simulink model "nano_distribution_distiller_controller_ver1"  (R2021a)
settings: Solver=VariableStepAuto  StartTime=0.0  StopTime=10.0  RelTol=1e-3
libraries: arduinolib x14
settings Model: Creator=Intuito_PC  LastModifiedBy=Intuito_PC

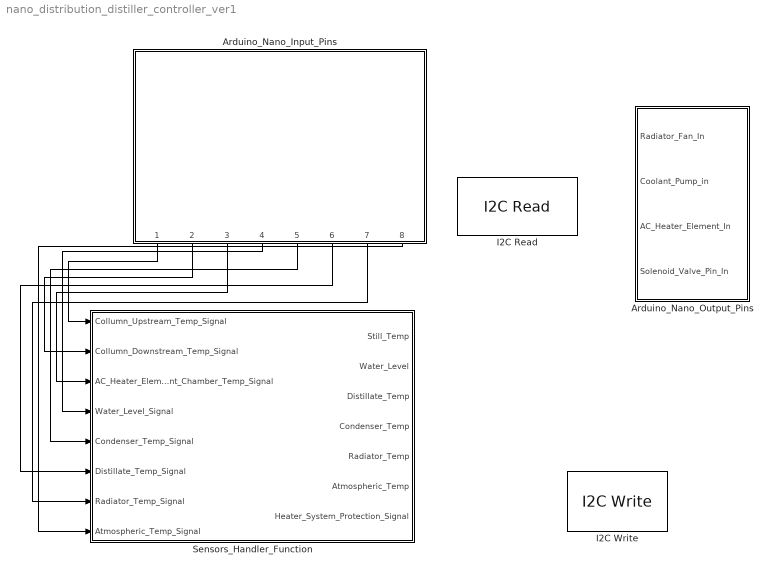
== system nano_distribution_distiller_controller_ver1 ==
  Arduino_Nano_Input_Pins : Subsystem
  Arduino_Nano_Output_Pins : Subsystem
  I2C Read : arduinolib/I2C Read  I2CModule=0  Mode=Master  SlaveAddress=10  SlaveByteOrder=BigEndian  Direction=Receiver  RegisterAddressMode=on  RegisterAddress=0  SlaveDataType=uint8  DataLength=1  NoAck=off  RepeatedStart=off  OutputStatus=off  blockPlatform=ARDUINO  SampleTime=0.25
      settings: SourceProductBaseCode=ARDUINO
  I2C Write : arduinolib/I2C Write  I2CModule=0  Mode=Master  SlaveAddress=10  SlaveByteOrder=BigEndian  Direction=Transmitter  RegisterAddressMode=on  RegisterAddress=0  SlaveDataType=uint8  DataLength=1  NoAck=off  RepeatedStart=off  OutputStatus=off  blockPlatform=ARDUINO
      settings: SourceProductBaseCode=ARDUINO
  Sensors_Handler_Function : Subsystem
  wires:
  Arduino_Nano_Input_Pins/8(Atmospheric_Temp_Signal) -> Sensors_Handler_Function/8(Atmospheric_Temp_Signal)
  Arduino_Nano_Input_Pins/7(Radiator_Temp_Signal) -> Sensors_Handler_Function/7(Radiator_Temp_Signal)
  Arduino_Nano_Input_Pins/3(AC_Heater_Element_Chamber_Temp_Signal) -> Sensors_Handler_Function/3(AC_Heater_Element_Chamber_Temp_Signal)
  Arduino_Nano_Input_Pins/1(Collumn_Upstream_Temp_Signal) -> Sensors_Handler_Function/1(Collumn_Upstream_Temp_Signal)
  Arduino_Nano_Input_Pins/2(Collumn_Downstream_Temp_Signal) -> Sensors_Handler_Function/2(Collumn_Downstream_Temp_Signal)
  Arduino_Nano_Input_Pins/6(Distillate_Temp_Signal) -> Sensors_Handler_Function/6(Distillate_Temp_Signal)
  Arduino_Nano_Input_Pins/5(Condenser_Temp_Signal) -> Sensors_Handler_Function/5(Condenser_Temp_Signal)
  Arduino_Nano_Input_Pins/4(Water_Level_Signal) -> Sensors_Handler_Function/4(Water_Level_Signal)

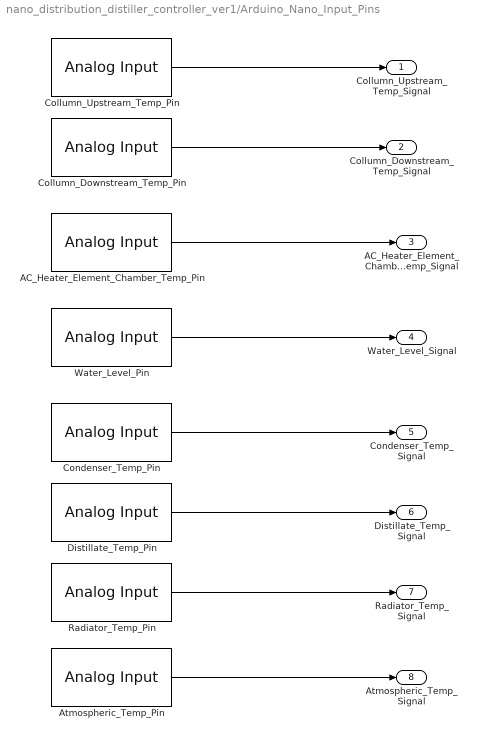
== system nano_distribution_distiller_controller_ver1/Arduino_Nano_Input_Pins ==
  AC_Heater_Element_Chamber_Temp_Pin : arduinolib/Analog Input  pinNumber=4  ReadResultsOnly=off  ConversionTriggerSource=Software  ExternalTriggerType=uint32( 0 )  OutputDataType=uint16  EnableConversionCompleteNotify=off  EnableOuputStatus=off  SampleTime=-1  blockPlatform=arduino
  Atmospheric_Temp_Pin : arduinolib/Analog Input  pinNumber=4  ReadResultsOnly=off  ConversionTriggerSource=Software  ExternalTriggerType=uint32( 0 )  OutputDataType=uint16  EnableConversionCompleteNotify=off  EnableOuputStatus=off  SampleTime=-1  blockPlatform=arduino
  Collumn_Downstream_Temp_Pin : arduinolib/Analog Input  pinNumber=4  ReadResultsOnly=off  ConversionTriggerSource=Software  ExternalTriggerType=uint32( 0 )  OutputDataType=uint16  EnableConversionCompleteNotify=off  EnableOuputStatus=off  SampleTime=-1  blockPlatform=arduino
  Collumn_Upstream_Temp_Pin : arduinolib/Analog Input  pinNumber=4  ReadResultsOnly=off  ConversionTriggerSource=Software  ExternalTriggerType=uint32( 0 )  OutputDataType=uint16  EnableConversionCompleteNotify=off  EnableOuputStatus=off  SampleTime=-1  blockPlatform=arduino
  Condenser_Temp_Pin : arduinolib/Analog Input  pinNumber=4  ReadResultsOnly=off  ConversionTriggerSource=Software  ExternalTriggerType=uint32( 0 )  OutputDataType=uint16  EnableConversionCompleteNotify=off  EnableOuputStatus=off  SampleTime=-1  blockPlatform=arduino
  Distillate_Temp_Pin : arduinolib/Analog Input  pinNumber=4  ReadResultsOnly=off  ConversionTriggerSource=Software  ExternalTriggerType=uint32( 0 )  OutputDataType=uint16  EnableConversionCompleteNotify=off  EnableOuputStatus=off  SampleTime=-1  blockPlatform=arduino
  Radiator_Temp_Pin : arduinolib/Analog Input  pinNumber=4  ReadResultsOnly=off  ConversionTriggerSource=Software  ExternalTriggerType=uint32( 0 )  OutputDataType=uint16  EnableConversionCompleteNotify=off  EnableOuputStatus=off  SampleTime=-1  blockPlatform=arduino
  Water_Level_Pin : arduinolib/Analog Input  pinNumber=4  ReadResultsOnly=off  ConversionTriggerSource=Software  ExternalTriggerType=uint32( 0 )  OutputDataType=uint16  EnableConversionCompleteNotify=off  EnableOuputStatus=off  SampleTime=-1  blockPlatform=arduino
  Collumn_Upstream_Temp_Signal : Outport
  Collumn_Downstream_Temp_Signal : Outport  Port=2
  AC_Heater_Element_Chamber_Temp_Signal : Outport  Port=3
  Water_Level_Signal : Outport  Port=4
  Condenser_Temp_Signal : Outport  Port=5
  Distillate_Temp_Signal : Outport  Port=6
  Radiator_Temp_Signal : Outport  Port=7
  Atmospheric_Temp_Signal : Outport  Port=8
  wires:
  Collumn_Upstream_Temp_Pin/1 -> Collumn_Upstream_Temp_Signal/1
  Collumn_Downstream_Temp_Pin/1 -> Collumn_Downstream_Temp_Signal/1
  AC_Heater_Element_Chamber_Temp_Pin/1 -> AC_Heater_Element_Chamber_Temp_Signal/1
  Water_Level_Pin/1 -> Water_Level_Signal/1
  Condenser_Temp_Pin/1 -> Condenser_Temp_Signal/1
  Distillate_Temp_Pin/1 -> Distillate_Temp_Signal/1
  Radiator_Temp_Pin/1 -> Radiator_Temp_Signal/1
  Atmospheric_Temp_Pin/1 -> Atmospheric_Temp_Signal/1

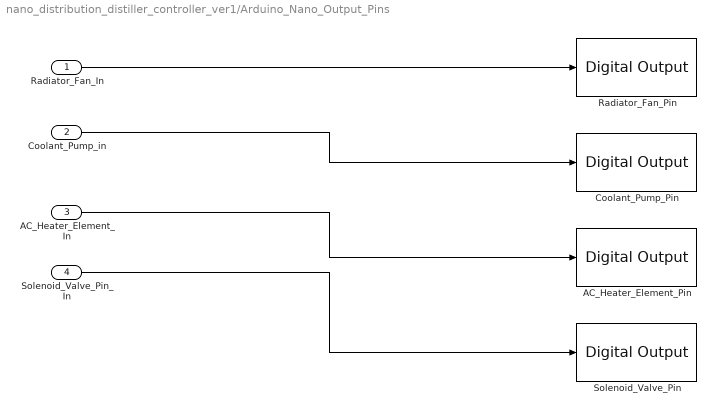
== system nano_distribution_distiller_controller_ver1/Arduino_Nano_Output_Pins ==
  Radiator_Fan_In : Inport
  Coolant_Pump_in : Inport  Port=2
  AC_Heater_Element_In : Inport  Port=3
  Solenoid_Valve_Pin_In : Inport  Port=4
  AC_Heater_Element_Pin : arduinolib/Digital Output  pinNumber=5  Direction=output  blockPlatform=arduino
  Coolant_Pump_Pin : arduinolib/Digital Output  pinNumber=5  Direction=output  blockPlatform=arduino
  Radiator_Fan_Pin : arduinolib/Digital Output  pinNumber=5  Direction=output  blockPlatform=arduino
  Solenoid_Valve_Pin : arduinolib/Digital Output  pinNumber=5  Direction=output  blockPlatform=arduino
  wires:
  Coolant_Pump_in/1 -> Coolant_Pump_Pin/1
  Radiator_Fan_In/1 -> Radiator_Fan_Pin/1
  Solenoid_Valve_Pin_In/1 -> Solenoid_Valve_Pin/1
  AC_Heater_Element_In/1 -> AC_Heater_Element_Pin/1

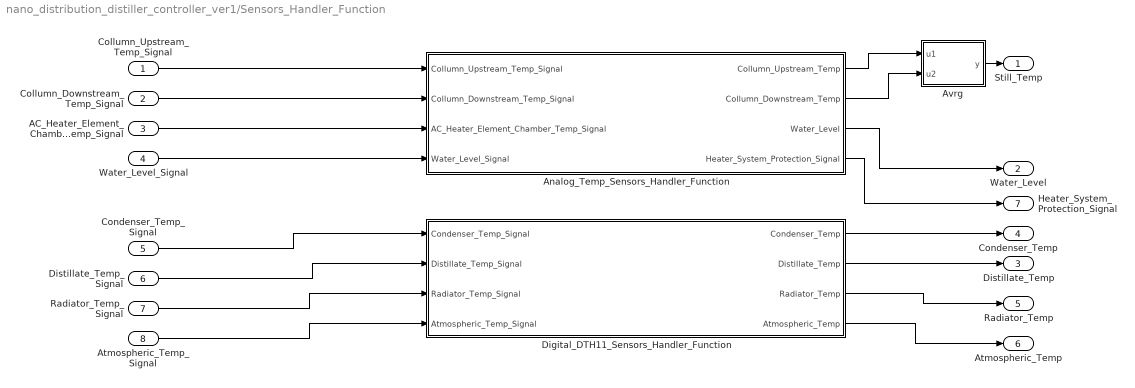
== system nano_distribution_distiller_controller_ver1/Sensors_Handler_Function ==
  Collumn_Upstream_Temp_Signal : Inport
  Collumn_Downstream_Temp_Signal : Inport  Port=2
  AC_Heater_Element_Chamber_Temp_Signal : Inport  Port=3
  Water_Level_Signal : Inport  Port=4
  Condenser_Temp_Signal : Inport  Port=5
  Distillate_Temp_Signal : Inport  Port=6
  Radiator_Temp_Signal : Inport  Port=7
  Atmospheric_Temp_Signal : Inport  Port=8
  Analog_Temp_Sensors_Handler_Function : MATLAB Function  TreatAsAtomicUnit=on
  Avrg : MATLAB Function  TreatAsAtomicUnit=on
  Digital_DTH11_Sensors_Handler_Function : MATLAB Function  TreatAsAtomicUnit=on
  Still_Temp : Outport
  Water_Level : Outport  Port=2
  Distillate_Temp : Outport  Port=3
  Condenser_Temp : Outport  Port=4
  Radiator_Temp : Outport  Port=5
  Atmospheric_Temp : Outport  Port=6
  Heater_System_Protection_Signal : Outport  Port=7
  wires:
  Condenser_Temp_Signal/1 -> Digital_DTH11_Sensors_Handler_Function/1(Condenser_Temp_Signal)
  Distillate_Temp_Signal/1 -> Digital_DTH11_Sensors_Handler_Function/2(Distillate_Temp_Signal)
  Radiator_Temp_Signal/1 -> Digital_DTH11_Sensors_Handler_Function/3(Radiator_Temp_Signal)
  Atmospheric_Temp_Signal/1 -> Digital_DTH11_Sensors_Handler_Function/4(Atmospheric_Temp_Signal)
  Water_Level_Signal/1 -> Analog_Temp_Sensors_Handler_Function/4(Water_Level_Signal)
  AC_Heater_Element_Chamber_Temp_Signal/1 -> Analog_Temp_Sensors_Handler_Function/3(AC_Heater_Element_Chamber_Temp_Signal)
  Collumn_Downstream_Temp_Signal/1 -> Analog_Temp_Sensors_Handler_Function/2(Collumn_Downstream_Temp_Signal)
  Collumn_Upstream_Temp_Signal/1 -> Analog_Temp_Sensors_Handler_Function/1(Collumn_Upstream_Temp_Signal)
  Digital_DTH11_Sensors_Handler_Function/1(Condenser_Temp) -> Condenser_Temp/1
  Digital_DTH11_Sensors_Handler_Function/2(Distillate_Temp) -> Distillate_Temp/1
  Digital_DTH11_Sensors_Handler_Function/3(Radiator_Temp) -> Radiator_Temp/1
  Digital_DTH11_Sensors_Handler_Function/4(Atmospheric_Temp) -> Atmospheric_Temp/1
  Analog_Temp_Sensors_Handler_Function/3(Water_Level) -> Water_Level/1
  Analog_Temp_Sensors_Handler_Function/4(Heater_System_Protection_Signal) -> Heater_System_Protection_Signal/1
  Avrg/1(y) -> Still_Temp/1
  Analog_Temp_Sensors_Handler_Function/1(Collumn_Upstream_Temp) -> Avrg/1(u1)
  Analog_Temp_Sensors_Handler_Function/2(Collumn_Downstream_Temp) -> Avrg/2(u2)

== matlab function nano_distribution_distiller_controller_ver1/Sensors_Handler_Function/Analog_Temp_Sensors_Handler_Function ==
  data: Collumn_Upstream_Temp_Signal input; Collumn_Upstream_Temp output; Collumn_Downstream_Temp_Signal input; AC_Heater_Element_Chamber_Temp_Signal input; Water_Level_Signal input; Collumn_Downstream_Temp output; Water_Level output; Heater_System_Protection_Signal output
function [Collumn_Upstream_Temp, Collumn_Downstream_Temp, Water_Level, Heater_System_Protection_Signal] = fcn(Collumn_Upstream_Temp_Signal, Collumn_Downstream_Temp_Signal, AC_Heater_Element_Chamber_Temp_Signal, Water_Level_Signal)
% Analog Temp Sensors Constants
THERMISTORNOMINAL = 90000;
TEMPERATURENOMINAL = 298; % 25 dge_C
BCOEFFICIENT = 3950;
SERIESRESISTOR = 10000; % R_1

% Temp sensor 1
R_1 = double(SERIESRESISTOR*(Collumn_Upstream_Temp_Signal/1023)/(5 - (Collumn_Upstream_Temp_Signal/1023)*4.99)); % NTC Resistance
Collumn_Upstream_Temp = 1/(1/TEMPERATURENOMINAL - log(abs(THERMISTORNOMINAL/R_1))/BCOEFFICIENT) -273; % Compute temp
% Temp sensor 2
R_2 = double(SERIESRESISTOR*(Collumn_Downstream_Temp_Signal/1023)/(5 - (Collumn_Downstream_Temp_Signal/1023)*4.99)); % NTC Resistance
Collumn_Downstream_Temp = 1/(1/TEMPERATURENOMINAL - log(abs(THERMISTORNOMINAL/R_2))/BCOEFFICIENT) -273; % Compute temp
% Temp sensor 3
R_3 = double(SERIESRESISTOR*(AC_Heater_Element_Chamber_Temp_Signal/1023)/(5 - (AC_Heater_Element_Chamber_Temp_Signal/1023)*4.99)); % NTC Resistance
AC_Heater_Element_Chamber_Temp = 1/(1/TEMPERATURENOMINAL - log(abs(THERMISTORNOMINAL/R_3))/BCOEFFICIENT) -273; % Compute temp

% Water level sensor
Water_Level = double(Water_Level_Signal/1023*100);

% Heater System Protection
if AC_Heater_Element_Chamber_Temp > 160
    Heater_System_Protection_Signal = 1;
else
    Heater_System_Protection_Signal = 0;
end
end

== matlab function nano_distribution_distiller_controller_ver1/Sensors_Handler_Function/Digital_DTH11_Sensors_Handler_Function ==
  data: Condenser_Temp_Signal input; Condenser_Temp output; Distillate_Temp_Signal input; Radiator_Temp_Signal input; Atmospheric_Temp_Signal input; Distillate_Temp output; Radiator_Temp output; Atmospheric_Temp output
function [Condenser_Temp, Distillate_Temp, Radiator_Temp, Atmospheric_Temp] = fcn(Condenser_Temp_Signal, Distillate_Temp_Signal, Radiator_Temp_Signal, Atmospheric_Temp_Signal)
% Analog Temp Sensors Constants
THERMISTORNOMINAL = 90000;
TEMPERATURENOMINAL = 298; % 25 dge_C
BCOEFFICIENT = 3950;
SERIESRESISTOR = 10000; % R_1

% Temp sensor 1
R_1 = double(SERIESRESISTOR*(Condenser_Temp_Signal/1023)/(5 - (Condenser_Temp_Signal/1023)*4.99)); % NTC Resistance
Condenser_Temp = 1/(1/TEMPERATURENOMINAL - log(abs(THERMISTORNOMINAL/R_1))/BCOEFFICIENT) -273; % Compute temp
% Temp sensor 2
R_2 = double(SERIESRESISTOR*(Distillate_Temp_Signal/1023)/(5 - (Distillate_Temp_Signal/1023)*4.99)); % NTC Resistance
Distillate_Temp = 1/(1/TEMPERATURENOMINAL - log(abs(THERMISTORNOMINAL/R_2))/BCOEFFICIENT) -273; % Compute temp
% Temp sensor 3
R_3 = double(SERIESRESISTOR*(Radiator_Temp_Signal/1023)/(5 - (Radiator_Temp_Signal/1023)*4.99)); % NTC Resistance
Radiator_Temp = 1/(1/TEMPERATURENOMINAL - log(abs(THERMISTORNOMINAL/R_3))/BCOEFFICIENT) -273; % Compute temp
% Temp sensor 4
R_4 = double(SERIESRESISTOR*(Atmospheric_Temp_Signal/1023)/(5 - (Atmospheric_Temp_Signal/1023)*4.99)); % NTC Resistance
Atmospheric_Temp = 1/(1/TEMPERATURENOMINAL - log(abs(THERMISTORNOMINAL/R_4))/BCOEFFICIENT) -273; % Compute temp
end

== matlab function nano_distribution_distiller_controller_ver1/Sensors_Handler_Function/Avrg ==
  data: u1 input; y output; u2 input
function y = fcn(u1, u2)
% Average
y = (u1 + u2)/2;
end
